simulink model "Piper_ident_sol"  (R2023b)
settings: Solver=ode3  StartTime=0.0  StopTime=200  FixedStep=0.01  RelTol=1e-3
values from neighbouring files (symbols this model uses):
  omegas = [ omega_low , omega_mid , omega_high ]    [Piper_ident_par_sol.m]
  phis = 2*pi*rand(1,length(omegas))    [Piper_ident_par_sol.m]
undefined symbols (not defined in the file or in its folder): denP, numP
settings Model: Creator=jerome  LastModifiedBy=jerome
settings ModelReferenceCC: EnableRefExpFcnMdlSchedulingChecks=on

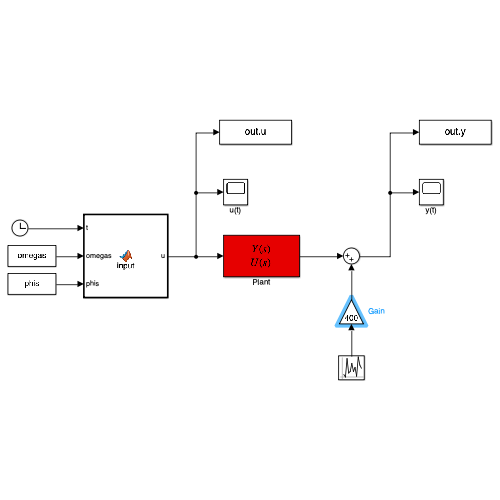
[thumbnail: Simulink's stored preview of the top-level diagram]
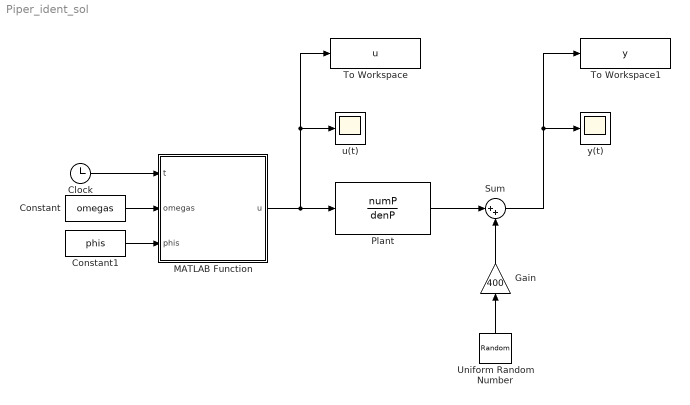
== system Piper_ident_sol ==
  Clock : Clock
  Constant : Constant  Value=omegas  VectorParams1D=off
  Constant1 : Constant  Value=phis  VectorParams1D=off
  Gain : Gain  Gain=400
  MATLAB Function : MATLAB Function  TreatAsAtomicUnit=on
  Plant : TransferFcn  Numerator=numP  Denominator=denP
  Sum : Sum  Inputs=|++
  To Workspace : ToWorkspace  VariableName=u  SampleTime=-1
  To Workspace1 : ToWorkspace  VariableName=y  SampleTime=-1
  Uniform Random Number : UniformRandomNumber  SampleTime=0.01
  u(t) : Scope
  y(t) : Scope
  wires:
  MATLAB Function/1(u) -> To Workspace/1, u(t)/1, Plant/1
  Clock/1 -> MATLAB Function/1(t)
  Constant/1 -> MATLAB Function/2(omegas)
  Constant1/1 -> MATLAB Function/3(phis)
  Plant/1 -> Sum/1
  Uniform Random Number/1 -> Gain/1
  Sum/1 -> To Workspace1/1, y(t)/1
  Gain/1 -> Sum/2

== matlab function Piper_ident_sol/MATLAB Function ==
  data: t input; u output; omegas input; phis input
function u = input(t,omegas,phis)

u = sum( sin(omegas*t + phis) );
